simulink model "Melo"  (Simulink 6.5)
settings: Solver=FixedStepDiscrete  SolverMode=SingleTasking  StartTime=0.0  StopTime=3  RelTol=1e-3
InitFcn:
  | Ts=2e-6; load power_acdrive_init;
undefined symbols (not defined in the file): DiscIntNeverNeededParam, powergui
libraries: powerlib x13, simulink x2
Description:
  | The Model initialization function Callback automatically
  | 
  | sets the sample time  to 2e-6 sec.  and loads the initial
  | 
  | states vector xInitial. The initial state vector is saved in the
  | 
  | power_acdrive_init.mat file.
  | 
  | 
  | 
  | Check  the Initial state checkbox in the Simulation
  | 
  | parameters/Workspace I/O to start in steady state with a
  | 
  | speed of 120 rad/s and a torque of 0 N.m/s,
settings Model: Creator=Hoang Lehuy, Laval University  LastModifiedBy=RS  ExtModeTrigMode=oneshot  ExtModeArmWhenConnect=off  ExtModeAutoUpdateStatusClock=off
settings DataIOCC: LimitDataPoints=off  SaveFinalState=on  SaveOutput=off  SaveTime=off  SignalLoggingName=sigsOut
settings OptimizationCC: BlockReduction=off  InlineInvariantSignals=on
settings DebuggingCC: CheckExecutionContextPreStartOutputMsg=on  CheckExecutionContextRuntimeOutputMsg=on  SolverPrmCheckMsg=none  MultiTaskDSMMsg=warning  MultiTaskCondExecSysMsg=none  UnconnectedOutputMsg=none  StrictBusMsg=None
settings HardwareCC: TargetUnknown=on
settings RTWCC: IncludeERTFirstTime=on

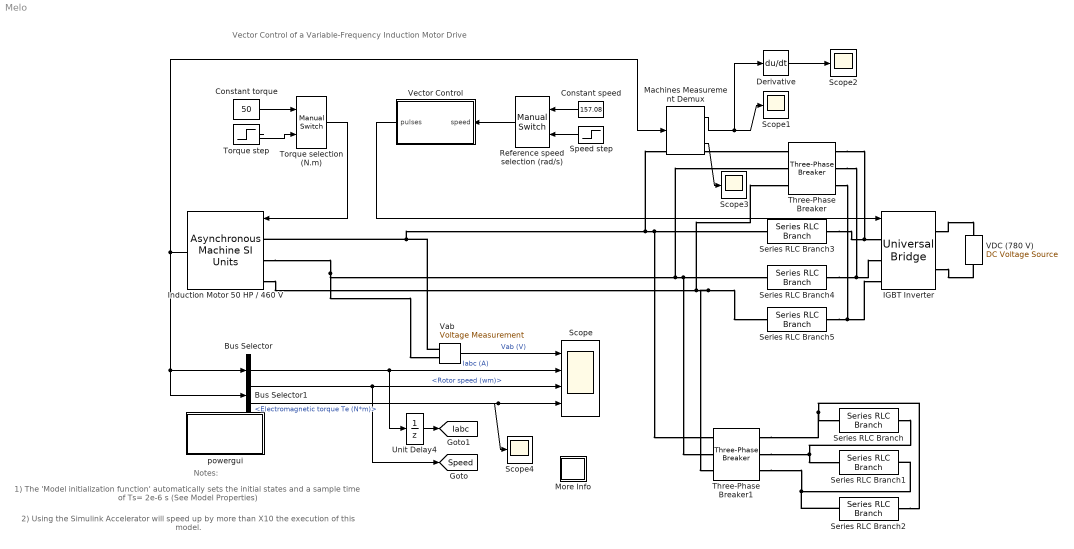
== system Melo ==
  note: Vector Control of a Variable-Frequency Induction Motor Drive
  note: 2) Using the Simulink Accelerator will speed up by more
      |      than X10 the execution of this model.
  note: 1) The 'Model initialization function' automatically sets  the initial states
      |     and a sample time of Ts= 2e-6 s  (See Model Properties)
  note: Notes:
  Bus Selector : BusSelector  OutputSignals=Stator measurements.Stator current is_a (A),Stator measurements.Stator current is_b (A),Stator measurements.Stator current is_c (A)  OutputAsBus=on
  Bus Selector1 : BusSelector  OutputSignals=Mechanical.Rotor speed (wm),Mechanical.Electromagnetic torque Te (N*m)
  Constant speed : Constant  Orientation=left  Value=157.08  OutDataType=sfix(16)  ConRadixGroup=Use specified scaling  OutScaling=2^0  SampleTime=inf  FramePeriod=inf
  Constant torque : Constant  Value=50  OutDataType=sfix(16)  ConRadixGroup=Use specified scaling  OutScaling=2^0  SampleTime=inf  FramePeriod=inf
  Derivative : Derivative
  IGBT Inverter : powerlib/Power Electronics/Universal Bridge  DialogController=PMDialogs.PMDefaultMaskDlg  SystemSampleTime=-1  Arms=3  SnubberResistance=1000  SnubberCapacitance=inf  Device=IGBT / Diodes  Ron=1e-3  Lon=0  ForwardVoltages="[  0.8  0.8  ]"  ForwardVoltage=.8  GTOparameters=[ 1e-6 , 1e-6 ]  IGBTparameters=[ 1e-6 , 2e-6 ]  Measurements=None  converterType=Rectifier
  Induction Motor 50 HP / 460 V : powerlib/Machines/Asynchronous Machine SI Units  Orientation=left  DialogController=PMDialogs.PMDefaultMaskDlg  SystemSampleTime=-1  PresetModel=No  MechanicalLoad=Torque Tm  ShowDetailedParameters=on  RotorType=Squirrel-cage  ReferenceFrame=Stationary  NominalParameters=[ 50*746, 460, 60 ]  Stator=[ 0.087 0.8e-3 ]  Rotor="[ 0.228  0.8e-3 ]"  Lm=34.7e-3  Mechanical="[1.662  0.1 2 ]"  PolePairs=2  InitialConditions="[ 1, 0 ,  0 , 0 , 0 , 0 , 0 , 0 ]"  Units=1  LoadFlowParameters=0  SimulateSaturation=off  Saturation=[0 0;0 0]
  Machines Measurement Demux : powerlib/Machines/Machines Measurement Demux  DialogController=PMDialogs.PMDefaultMaskDlg  SystemSampleTime=-1  machType=Asynchronous  ssm1=on  ssm2=on  ssm3=on  ssm4=on  ssm5=on  ssm6=on  sm1=off  sm2=off  sm3=off  sm4=off  sm5=off  sm6=off  sm7=off  sm8=on  sm9=off  sm10=off  sm11=off  sm115=off  sm12=off  sm13=off  sm14=off  asm1=off  asm2=off  asm3=off  asm4=off  asm5=off  asm6=off  asm7=on  asm8=on  asm9=off  asm10=off  asm11=off  pmsm1=on  pmsm2=on  pmsm3=on  pmsm4=off  pmsm5=on  pmsm6=on  pmsm7=on  lastType=1
  More Info : Subsystem
      settings: OpenFcn=showdemo(bdroot(gcb))
      mask Display: disp('?')
  Reference speed selection (rad/s) : simulink/Signal Routing/Manual Switch  Orientation=left  SystemSampleTime=-1  sw=1  action=0
  Scope : Scope  NumInputPorts=4
      settings: TimeRange=3  YMin=-1000~-500~0~-100  YMax=1000~500~200~400  Decimation=20  SampleTime=5e-6
  Scope{1..4} (4 alike) : Scope
      Scope1 settings: Decimation=20
      Scope2 settings: SaveName=ScopeData2  Decimation=20
      Scope3 settings: SaveName=ScopeData3  Decimation=20
      Scope4 settings: SaveName=ScopeData4  MaxDataPoints=10000000  Decimation=20
  Series RLC Branch : powerlib/Elements/Series RLC Branch  DialogController=PMDialogs.PMDefaultMaskDlg  PhysicalDomain=powersysdomain  SubClassName=unknown  LeftPortType=p1  RightPortType=p1  LConnTagsString=__new0  RConnTagsString=__new0  BranchType=C  Resistance=1  Inductance=1e-3  SetiL0=off  InitialCurrent=0  Capacitance=1e-3  Setx0=off  InitialVoltage=0  Measurements=None
  Series RLC Branch1 : powerlib/Elements/Series RLC Branch  DialogController=PMDialogs.PMDefaultMaskDlg  PhysicalDomain=powersysdomain  SubClassName=unknown  LeftPortType=p1  RightPortType=p1  LConnTagsString=__new0  RConnTagsString=__new0  BranchType=C  Resistance=1  Inductance=1e-3  SetiL0=off  InitialCurrent=0  Capacitance=1e-3  Setx0=off  InitialVoltage=0  Measurements=None
  Series RLC Branch2 : powerlib/Elements/Series RLC Branch  DialogController=PMDialogs.PMDefaultMaskDlg  PhysicalDomain=powersysdomain  SubClassName=unknown  LeftPortType=p1  RightPortType=p1  LConnTagsString=__new0  RConnTagsString=__new0  BranchType=C  Resistance=1  Inductance=1e-3  SetiL0=off  InitialCurrent=0  Capacitance=1e-3  Setx0=off  InitialVoltage=0  Measurements=None
  Series RLC Branch3 : powerlib/Elements/Series RLC Branch  DialogController=PMDialogs.PMDefaultMaskDlg  PhysicalDomain=powersysdomain  SubClassName=unknown  LeftPortType=p1  RightPortType=p1  LConnTagsString=__new0  RConnTagsString=__new0  BranchType=R  Resistance=3  Inductance=1e-3  SetiL0=off  InitialCurrent=0  Capacitance=1e-6  Setx0=off  InitialVoltage=0  Measurements=None
  Series RLC Branch4 : powerlib/Elements/Series RLC Branch  DialogController=PMDialogs.PMDefaultMaskDlg  PhysicalDomain=powersysdomain  SubClassName=unknown  LeftPortType=p1  RightPortType=p1  LConnTagsString=__new0  RConnTagsString=__new0  BranchType=R  Resistance=3  Inductance=1e-3  SetiL0=off  InitialCurrent=0  Capacitance=1e-6  Setx0=off  InitialVoltage=0  Measurements=None
  Series RLC Branch5 : powerlib/Elements/Series RLC Branch  DialogController=PMDialogs.PMDefaultMaskDlg  PhysicalDomain=powersysdomain  SubClassName=unknown  LeftPortType=p1  RightPortType=p1  LConnTagsString=__new0  RConnTagsString=__new0  BranchType=R  Resistance=3  Inductance=1e-3  SetiL0=off  InitialCurrent=0  Capacitance=1e-6  Setx0=off  InitialVoltage=0  Measurements=None
  Speed step : Step  Orientation=left  Time=0.2  Before=120  After=160  SampleTime=0
  Three-Phase Breaker : powerlib/Elements/Three-Phase Breaker  DialogController=PMDialogs.PMDefaultMaskDlg  SystemSampleTime=-1  InitialState=closed  SwitchA=on  SwitchB=on  SwitchC=on  SwitchTimes=0  External=off  BreakerResistance=0.001  SnubberResistance=1e6  SnubberCapacitance=inf  Measurements=None
  Three-Phase Breaker1 : powerlib/Elements/Three-Phase Breaker  DialogController=PMDialogs.PMDefaultMaskDlg  SystemSampleTime=-1  InitialState=open  SwitchA=on  SwitchB=on  SwitchC=on  SwitchTimes=0  External=off  BreakerResistance=0.001  SnubberResistance=1e6  SnubberCapacitance=inf  Measurements=None
  Torque selection (N.m) : simulink/Signal Routing/Manual Switch  SystemSampleTime=-1  sw=0  action=0
  Torque step : Step  Time=1.8  After=50  SampleTime=0
  Unit Delay4 : UnitDelay  SampleTime=Ts
  VDC (780 V) : powerlib/Electrical Sources/DC Voltage Source  Description=source block  Orientation=up  DialogController=PMDialogs.PMDefaultMaskDlg  SystemSampleTime=-1  Amplitude=780  Measurements=None
      settings: AttributesFormatString=\n
  Vab : powerlib/Measurements/Voltage Measurement  Tag=PoWeRsYsTeMmEaSuReMeNt  DialogController=PMDialogs.PMDefaultMaskDlg  SystemSampleTime=-1  PhasorSimulation=off  OutputType=Magnitude  PSBequivalent=0
  Vector Control : Subsystem  Orientation=left
  powergui : Subsystem  Priority=2  AncestorBlock=powerlib/powergui  InitFcn=powergui( 'InitFcn_Callback' , gcb , 0 , [ ] );  mask(PSB option menu block){SimulationMode=Discrete, SampleTime=Ts, echomessages=off, RestoreLinks=warning, x0status=blocks, Frange=[0:2:500], Ylog=off, Xlog=on, ShowGrid=off, save=off, variable=ZData, structure=ScopeData4, ZoomFFT=on, StartTime=2.8, cycles=10, DisplayStyle=2, fundamental=100, FreqAxis=off, MaxFrequency=1000, frequencyindice=60, frequencyindicesteady=1, RmsSteady=1, display=off, Ts=0, frequency=60, methode=off, HookPort=off, Interpol=off}
      mask prompts: SimulationMode "Simulation mode"; SampleTime "Sample time Ts (when simulation mode is Discrete) (s)"; echomessages "Echo  Messages"; RestoreLinks "Restore disabled links"; x0status "Initial electrical states status"; Frange "Impedance tool: Frequency Range"; Ylog "Impedance tool: Log impedance"; Xlog "Impedance tool: log Frequency"; ShowGrid "Impedance tool: grid"; save "Impedance tool: Save Data To Workspace"; variable "Impedance tool: Variable Name"; structure "Structure Name (PSBFFTSCOPE)"; ZoomFFT "ZoomFFT (PSBFFTSCOPE)"; StartTime "Start Time (PSBFFTSCOPE)"; cycles "Cycles (PSBFFTSCOPE)"; DisplayStyle "Display style (PSBFFTSCOPE)"; fundamental "Fundamental (PSBFFTSCOPE)"; FreqAxis "Frequency Axis (PSBFFTSCOPE)"; MaxFrequency "Max Frequency (PSBFFTSCOPE)"; frequencyindice "Load flow frequency (Hz)"; frequencyindicesteady "Frequency indice (STEADYSTATE)"; RmsSteady "RMS display (STEADYSTATE)"; display "Display Results"; Ts "OBSOLETE 1"; frequency "Phasor frequency (Hz)"; methode "Phasor simulation"; HookPort "Hook port"; Interpol "Interpolate"
      mask init:
      | powerlibroot = which('powersysdomain');
      | PSBroot = powerlibroot(1:end-16);
      | %
      | switch SimulationMode
      | 	case 1
      | 		message=sprintf('Continuous');
      | 	case 2
      |         SampleTimeeval=evalin('base',SampleTime,'NaN');
      |         if isnan(SampleTimeeval)
      |             message=sprintf('Warning !!,\nUndefined sample time');
      |         else
      |             message=sprintf('Discrete,\nTs = %.4g s.',SampleTimeeval);
      |         end
      | 	case 3
      | 		message=sprintf('Phasors');
      | end
      | if strcmp(bdroot,'powerlib')
      |   message='powergui';
      | end
      | power_initmask();
      settings: CopyFcn=powergui( 'Copy_Callback' , gcb , 0 , [ ] );  ModelCloseFcn=powergui( 'CloseButton_Callback' , gcb , [ ] , [ ] );  PreSaveFcn=powergui( 'CloseButton_Callback' , gcb , [ ] , [ ] );  NameChangeFcn=powergui( 'NameChangeFcn_Callback' , gcb , 0 , [ ] );
      settings: DeleteFcn=|
      | powergui( 'Copy_Callback' , gcb , 1 , [ ] );
      | powergui( 'CloseButton_Callback' , gcb , [ ] , [ ] );
      settings: OpenFcn=|
      | if (power_openblockproxy ('secondary'))
      | powergui(gcb,'PM')
      | end;
      mask Help: web(psbhelp)
      mask StyleString: popup(Continuous|Discrete|Phasor),edit,checkbox,popup(yes|warning|no),popup(blocks|steady|zero),edit,checkbox,checkbox,checkbox,checkbox,edit,edit,checkbox,edit,edit,edit,edit,checkbox,edit,edit,edit,edit,checkbox,edit,edit,checkbox,checkbox,checkbox
      mask CallbackString: ||||||||||||||||||||||||||powergui('HookPort',[],[],gcb);|
      mask Display: disp(message)
  tag scope: Iabc=global, Speed=global
  wires:
  Bus Selector1/1 -> Scope/3, [Speed]  "<Rotor speed (wm)>"
  Vector Control/1(pulses) -> IGBT Inverter/1
  Torque step/1 -> Torque selection (N.m)/2
  Constant torque/1 -> Torque selection (N.m)/1
  Constant speed/1 -> Reference speed selection (rad/s)/1
  Speed step/1 -> Reference speed selection (rad/s)/2
  Bus Selector/1 -> Scope/2, Unit Delay4/1  "Iabc (A)"
  Vab/1 -> Scope/1  "Vab (V)"
  Bus Selector1/2 -> Scope/4, Scope4/1  "<Electromagnetic torque Te (N*m)>"
  Torque selection (N.m)/1 -> Induction Motor 50 HP / 460 V/1
  Reference speed selection (rad/s)/1 -> Vector Control/1(speed)
  Induction Motor 50 HP / 460 V/1 -> Bus Selector1/1, Bus Selector/1, Machines Measurement Demux/1
  Unit Delay4/1 -> [Iabc]
  Machines Measurement Demux/1 -> Scope1/1, Derivative/1
  Derivative/1 -> Scope2/1
  Machines Measurement Demux/2 -> Scope3/1
  connections:
  IGBT Inverter/RConn2 -- VDC (780 V)/LConn1
  IGBT Inverter/RConn1 -- VDC (780 V)/RConn1
  Series RLC Branch/RConn1 -- Series RLC Branch1/LConn1 -- Three-Phase Breaker1/RConn2
  Series RLC Branch2/RConn1 -- Series RLC Branch/LConn1 -- Three-Phase Breaker1/RConn1
  Series RLC Branch4/RConn1 -- IGBT Inverter/LConn2 -- Three-Phase Breaker/RConn2
  Series RLC Branch2/LConn1 -- Series RLC Branch1/RConn1 -- Three-Phase Breaker1/RConn3
  Vab/LConn1 -- Induction Motor 50 HP / 460 V/LConn1 -- Three-Phase Breaker/LConn1 -- Series RLC Branch3/LConn1 -- Three-Phase Breaker1/LConn1
  Induction Motor 50 HP / 460 V/LConn2 -- Vab/LConn2 -- Three-Phase Breaker/LConn2 -- Series RLC Branch4/LConn1 -- Three-Phase Breaker1/LConn2
  Induction Motor 50 HP / 460 V/LConn3 -- Three-Phase Breaker/LConn3 -- Series RLC Branch5/LConn1 -- Three-Phase Breaker1/LConn3
  Series RLC Branch5/RConn1 -- IGBT Inverter/LConn3 -- Three-Phase Breaker/RConn3
  Series RLC Branch3/RConn1 -- IGBT Inverter/LConn1 -- Three-Phase Breaker/RConn1

== system Melo/More Info ==
  note: H. Le-Huy (Universite Laval, Quebec)
  note: Case study : Variable-Frequency Induction Motor Drive
  note: Circuit Description
  note: Demonstration
  note: The induction motor is fed by a current-controlled PWM inverter which is built using a Universal Bridge block.
      | The motor drives a mechanical load characterized by inertia J, friction coeficient B, and load torque TL .
      | The speed control loop uses a proportional-integral controller to produce the quadrature-axis current reference
      | iq* which controls the motor torque.  The motor flux is controlled by the direct-axis current reference id*.
      | Block DQ-ABC is used to convert id* and iq* into current references ia*, ib*, and ic* for the current regulator.
      | Current and Voltage Measurement blocks provide signals for visualization purpose.
      | Motor current, speed, and torque signals are available at the output of the 'Asynchronous Machine' block.
  note: Motor starting
  note: Start the simulation. Observe the motor current, voltage, and speed during the starting on the scope.
      | At the end of the simulation time (3 s), the system has reached its steady-state.
  note: Response to a change in reference speed and load torque
  note: The initial conditions state vector `xInitial' to start with wm = 120 rad/s and TL = 0 N.m has been saved in the 'power_acdrive_init.mat'  file.
      | This file is automatically loaded in your  workspace when you start the simulation (see  Model Properties).
      | In order to use these initial conditions you have to enable them. Check the Simulation/Configuration Parameters menu ,
      | then select "Data Import/Export" and check "Initial state".
      |
      | Now, double click the two Manual Switch blocks to switch from  the  "Constant speed " and  "Constant torque" blocks to the Step blocks.
      | (Reference speed wref changed from 120 to 160 rad/s at t = 0.2 s and load torque changed from 0 to 200 N.m at  t= 1.8s).
      | Restart the simulation  and observe the drive response to successive changes in speed reference and load torque.

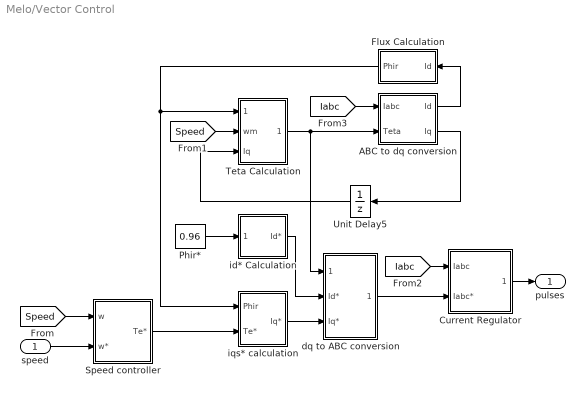
== system Melo/Vector Control ==
  speed : Inport
  ABC to dq conversion : Subsystem
  Current Regulator : Subsystem  mask(Regulateur de courant a hysteresis){h=20}
      mask prompts: h "Hysteresis band (A)"
  Flux Calculation : Subsystem  Orientation=left  mask(Flux Calcultation){}
      mask init:
      | NF=0.44572610323020e-6;
      | DF=[1 -0.99998715486734];
  Phir* : Constant  Value=0.96  OutDataType=sfix(16)  ConRadixGroup=Use specified scaling  OutScaling=2^0  SampleTime=inf  FramePeriod=inf
  Speed controller : Subsystem  mask(PI controller){Kp=13, Ki=26, Tlim=300, Ts=Ts}
      mask prompts: Kp "Proportional gain (Kp)"; Ki "Integral gain (Ki)"; Tlim "Torque limit (N.m)"; Ts "Sampling time (s)"
      mask help: Proportional-Integral Speed Controller
      mask Display: plot(0,0,100,100,[35,35,65],[70,30,30],[35,65],[45,60])
  Teta Calculation : Subsystem
  Unit Delay5 : UnitDelay  Orientation=left  SampleTime=Ts
  dq to ABC conversion : Subsystem
  id* Calculation : Subsystem
  iqs* calculation : Subsystem
  pulses : Outport
  wires:
  dq to ABC conversion/1(Iabc*) -> Current Regulator/2(Iabc*)
  Speed controller/1(Te*) -> iqs* calculation/2(Te*)
  Phir*/1 -> id* Calculation/1(Phir*)
  ABC to dq conversion/1(Id) -> Flux Calculation/1(Id)
  id* Calculation/1(Id*) -> dq to ABC conversion/2(Id*)
  Flux Calculation/1(Phir) -> Teta Calculation/1(Phir), iqs* calculation/1(Phir)
  ABC to dq conversion/2(Iq) -> Unit Delay5/1
  Unit Delay5/1 -> Teta Calculation/3(Iq)
  iqs* calculation/1(Iq*) -> dq to ABC conversion/3(Iq*)
  Teta Calculation/1(Teta) -> dq to ABC conversion/1(Teta), ABC to dq conversion/2(Teta)
  [Speed] -> Speed controller/1(w)
  [Speed] -> Teta Calculation/2(wm)
  [Iabc] -> Current Regulator/1(Iabc)
  [Iabc] -> ABC to dq conversion/1(Iabc)
  speed/1 -> Speed controller/2(w*)
  Current Regulator/1(Pulses) -> pulses/1

== system Melo/powergui ==
  note: Graphical user interface for the analysis of  SimPowerSystems circuits.
      | Place the Powergui block in the top-level of your model and double-click
      | on it to open the GUI.
  EquivalentModel1 : Subsystem
      mask init:
      | SPS = get_param(gcbh,'UserData');
      | if isempty(SPS)
      | 	Ts=1;
      |     A=0;
      |     B=0;
      |     C=0;
      |     D=0;
      |     x0=0;
      |     SwitchResistance=1;
      |     SwitchType=1;
      |     SwitchGateInitialValue=1;
      |     OutputsToResetToZero=1;
      | else
      | 	Ts=SPS.PowerguiInfo.Ts;
      | 	A=SPS.Adiscrete;
      |     B=SPS.Bdiscrete;
      |     C=SPS.Cdiscrete;
      |     D=SPS.Ddiscrete;
      |     x0=SPS.x0discrete;
      |     SwitchResistance=SPS.SwitchResistance;
      |     SwitchType=SPS.SwitchType;
      |     SwitchGateInitialValue=SPS.SwitchGateInitialValue;
      |     OutputsToResetToZero=SPS.YSwitchCurrent;
      | end
      mask Display:
      | color('orange')
      | disp('EQUIVALENT CIRCUIT')
  Ground : Ground
  Terminator : Terminator
  wires:
  Ground/1 -> Terminator/1

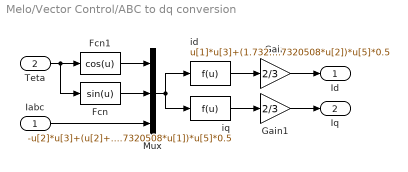
== system Melo/Vector Control/ABC to dq conversion ==
  Iabc : Inport
  Teta : Inport  Port=2
  Fcn : Fcn  Expr=sin(u)
  Fcn1 : Fcn  Expr=cos(u)
  Gain : Gain  Gain=2/3  SaturateOnIntegerOverflow=on
  Gain1 : Gain  Gain=2/3  SaturateOnIntegerOverflow=on
  Mux : Mux  Inputs=[1 1 3]
  id : Fcn  Expr=u[1]*u[3]+(1.7320508*u[2]-u[1])*u[4]*0.5+(-u[1]-1.7320508*u[2])*u[5]*0.5
  iq : Fcn  Expr=-u[2]*u[3]+(u[2]+1.7320508*u[1])*u[4]*0.5+(u[2]-1.7320508*u[1])*u[5]*0.5
  Id : Outport  InitialOutput=0
  Iq : Outport  Port=2  InitialOutput=0
  wires:
  Fcn/1 -> Mux/2
  Fcn1/1 -> Mux/1
  Teta/1 -> Fcn1/1, Fcn/1
  Mux/1 -> iq/1, id/1
  Iabc/1 -> Mux/3
  iq/1 -> Gain1/1
  id/1 -> Gain/1
  Gain/1 -> Id/1
  Gain1/1 -> Iq/1

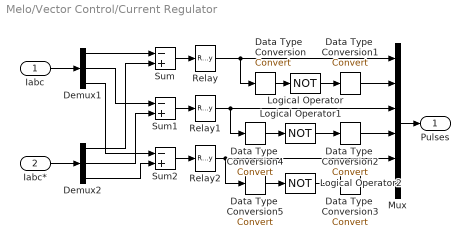
== system Melo/Vector Control/Current Regulator ==
  Iabc : Inport
  Iabc* : Inport  Port=2
  Data Type  Conversion : DataTypeConversion  OutDataTypeMode=boolean  SaturateOnIntegerOverflow=on  RndMeth=Zero
  Data Type  Conversion1 : DataTypeConversion  OutDataTypeMode=double  SaturateOnIntegerOverflow=on  RndMeth=Zero
  Data Type  Conversion2 : DataTypeConversion  OutDataTypeMode=double  SaturateOnIntegerOverflow=on  RndMeth=Zero
  Data Type  Conversion3 : DataTypeConversion  OutDataTypeMode=double  SaturateOnIntegerOverflow=on  RndMeth=Zero
  Data Type  Conversion4 : DataTypeConversion  OutDataTypeMode=boolean  SaturateOnIntegerOverflow=on  RndMeth=Zero
  Data Type  Conversion5 : DataTypeConversion  OutDataTypeMode=boolean  SaturateOnIntegerOverflow=on  RndMeth=Zero
  Demux1 : Demux  Outputs=3
  Demux2 : Demux  Outputs=3
  Logical Operator : Logic  Operator=NOT
  Logical Operator1 : Logic  Operator=NOT
  Logical Operator2 : Logic  Operator=NOT
  Mux : Mux  Inputs=6
  Relay : Relay  OnSwitchValue=h/2  OffSwitchValue=-h/2
  Relay1 : Relay  OnSwitchValue=h/2  OffSwitchValue=-h/2
  Relay2 : Relay  OnSwitchValue=h/2  OffSwitchValue=-h/2
  Sum : Sum  Inputs=-+  SaturateOnIntegerOverflow=on  InputSameDT=on
  Sum1 : Sum  Inputs=-+  SaturateOnIntegerOverflow=on  InputSameDT=on
  Sum2 : Sum  Inputs=-+  SaturateOnIntegerOverflow=on  InputSameDT=on
  Pulses : Outport  InitialOutput=0
  wires:
  Sum/1 -> Relay/1
  Sum1/1 -> Relay1/1
  Demux1/1 -> Sum/1
  Demux1/2 -> Sum1/1
  Mux/1 -> Pulses/1
  Iabc/1 -> Demux1/1
  Sum2/1 -> Relay2/1
  Demux1/3 -> Sum2/1
  Demux2/3 -> Sum2/2
  Demux2/2 -> Sum1/2
  Demux2/1 -> Sum/2
  Iabc*/1 -> Demux2/1
  Relay/1 -> Mux/1, Data Type  Conversion/1
  Relay1/1 -> Mux/3, Data Type  Conversion4/1
  Relay2/1 -> Mux/5, Data Type  Conversion5/1
  Data Type  Conversion/1 -> Logical Operator/1
  Logical Operator/1 -> Data Type  Conversion1/1
  Data Type  Conversion1/1 -> Mux/2
  Logical Operator1/1 -> Data Type  Conversion2/1
  Data Type  Conversion2/1 -> Mux/4
  Logical Operator2/1 -> Data Type  Conversion3/1
  Data Type  Conversion3/1 -> Mux/6
  Data Type  Conversion4/1 -> Logical Operator1/1
  Data Type  Conversion5/1 -> Logical Operator2/1

== system Melo/Vector Control/Flux Calculation ==
  note: Phir = Lm *Id / (1 +Tr .s)
  note: Lm = 34.7 mH
  note: Lr = Ll'r +Lm = 0.8 +34.7= 35.5 mH
  note: Tr = Lr / Rr = 0.1557 s
  note: Rr = 0.228 ohms
  Id : Inport  Orientation=left
  Discrete Tranfer Function : Subsystem  Orientation=left  mask(First Order Low Pass Filter (Discrete)){T=0.1557, Ts=Ts}
      mask prompts: T "Time constant T (s) :"; Ts "Time step (s)"
      mask help: H(s)=1/(1+T.s)
      mask init:
      | X=[0 1 2 3 4];
      |  Y=[-2 -2 -3 -4 -4];
      |  str=sprintf('\nH=1/(1+T.s)\n T= %g s\n\n\n',T);
      | num=1;
      | den=[T 1];
      | 
      | % discrete transfer function
      | % descending powers of z
      | numd= Ts/T;
      | dend=[ 1  (Ts-T)/T];
      mask Display:
      | plot(X,Y);
      | disp(str);
  Lm : Gain  Orientation=left  Gain=34.7e-3  SaturateOnIntegerOverflow=on
  Phir : Outport  Orientation=left
  wires:
  Discrete Tranfer Function/1(Out) -> Phir/1
  Id/1 -> Lm/1
  Lm/1 -> Discrete Tranfer Function/1(In)

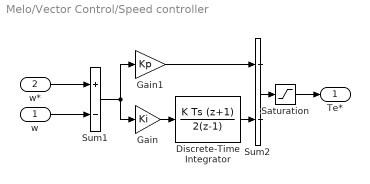
== system Melo/Vector Control/Speed controller ==
  w : Inport
  w* : Inport  Port=2
  Discrete-Time Integrator : DiscreteIntegrator  IntegratorMethod=Integration: Trapezoidal  SampleTime=Ts  LimitOutput=on  UpperSaturationLimit=Tlim  LowerSaturationLimit=-Tlim  ICPrevOutput=DiscIntNeverNeededParam  ICPrevScaledInput=DiscIntNeverNeededParam
  Gain : Gain  Gain=Ki  SaturateOnIntegerOverflow=on
  Gain1 : Gain  Gain=Kp  SaturateOnIntegerOverflow=on
  Saturation : Saturate  UpperLimit=Tlim  LowerLimit=-Tlim
  Sum1 : Sum  Inputs=+-  SaturateOnIntegerOverflow=on  InputSameDT=on
  Sum2 : Sum  SaturateOnIntegerOverflow=on  InputSameDT=on
  Te* : Outport  InitialOutput=0
  wires:
  Gain1/1 -> Sum2/1
  Gain/1 -> Discrete-Time Integrator/1
  Sum1/1 -> Gain/1, Gain1/1
  Discrete-Time Integrator/1 -> Sum2/2
  Sum2/1 -> Saturation/1
  Saturation/1 -> Te*/1
  w/1 -> Sum1/2
  w*/1 -> Sum1/1

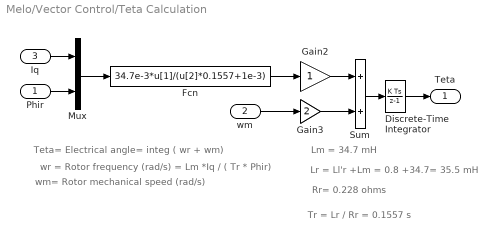
== system Melo/Vector Control/Teta Calculation ==
  note: Teta= Electrical angle= integ ( wr + wm)
  note: wr = Rotor frequency (rad/s) = Lm *Iq / ( Tr * Phir)
  note: Lm = 34.7 mH
  note: Rr= 0.228 ohms
  note: Lr = Ll'r +Lm = 0.8 +34.7= 35.5 mH
  note: wm= Rotor mechanical speed (rad/s)
  note: Tr = Lr / Rr = 0.1557 s
  Phir : Inport
  wm : Inport  Port=2
  Iq : Inport  Port=3
  Discrete-Time Integrator : DiscreteIntegrator  SampleTime=Ts  ICPrevOutput=DiscIntNeverNeededParam  ICPrevScaledInput=DiscIntNeverNeededParam
  Fcn : Fcn  Expr=34.7e-3*u[1]/(u[2]*0.1557+1e-3)
  Gain2 : Gain  SaturateOnIntegerOverflow=on
  Gain3 : Gain  Gain=2  SaturateOnIntegerOverflow=on
  Mux : Mux  Inputs=2
  Sum : Sum  SaturateOnIntegerOverflow=on  InputSameDT=on
  Teta : Outport  InitialOutput=0
  wires:
  Discrete-Time Integrator/1 -> Teta/1
  Sum/1 -> Discrete-Time Integrator/1
  Gain3/1 -> Sum/2
  Gain2/1 -> Sum/1
  wm/1 -> Gain3/1
  Fcn/1 -> Gain2/1
  Phir/1 -> Mux/2
  Iq/1 -> Mux/1
  Mux/1 -> Fcn/1

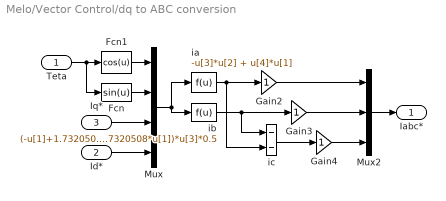
== system Melo/Vector Control/dq to ABC conversion ==
  Teta : Inport
  Id* : Inport  Port=2
  Iq* : Inport  Port=3
  Fcn : Fcn  Expr=sin(u)
  Fcn1 : Fcn  Expr=cos(u)
  Gain2 : Gain  SaturateOnIntegerOverflow=on
  Gain3 : Gain  SaturateOnIntegerOverflow=on
  Gain4 : Gain  SaturateOnIntegerOverflow=on
  Mux : Mux
  Mux2 : Mux  Inputs=3
  ia : Fcn  Expr=-u[3]*u[2] + u[4]*u[1]
  ib : Fcn  Expr=(-u[1]+1.7320508*u[2])*u[4]*0.5+(u[2]+1.7320508*u[1])*u[3]*0.5
  ic : Sum  Inputs=--  SaturateOnIntegerOverflow=on  InputSameDT=on
  Iabc* : Outport  InitialOutput=0
  wires:
  Fcn/1 -> Mux/2
  Fcn1/1 -> Mux/1
  Mux2/1 -> Iabc*/1
  Mux/1 -> ib/1, ia/1
  Teta/1 -> Fcn1/1, Fcn/1
  Iq*/1 -> Mux/3
  Id*/1 -> Mux/4
  Gain3/1 -> Mux2/2
  ic/1 -> Gain4/1
  Gain4/1 -> Mux2/3
  Gain2/1 -> Mux2/1
  ia/1 -> Gain2/1, ic/2
  ib/1 -> Gain3/1, ic/1

== system Melo/Vector Control/id* Calculation ==
  note: Id* = Phir*/ Lm
  note: Lm= 34.7 mH
  Phir* : Inport
  KF : Gain  Gain=1/34.7e-3  SaturateOnIntegerOverflow=on
  Id* : Outport
  wires:
  KF/1 -> Id*/1
  Phir*/1 -> KF/1

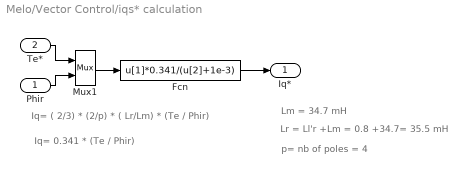
== system Melo/Vector Control/iqs* calculation ==
  note: Iq= ( 2/3) * (2/p) * ( Lr/Lm) * (Te / Phir)
  note: Lm = 34.7 mH
  note: Lr = Ll'r +Lm = 0.8 +34.7= 35.5 mH
  note: p= nb of poles = 4
  note: Iq= 0.341 * (Te / Phir)
  Phir : Inport
  Te* : Inport  Port=2
  Fcn : Fcn  Expr=u[1]*0.341/(u[2]+1e-3)
  Mux1 : Mux  Inputs=2
  Iq* : Outport  InitialOutput=0
  wires:
  Phir/1 -> Mux1/2
  Fcn/1 -> Iq*/1
  Te*/1 -> Mux1/1
  Mux1/1 -> Fcn/1

== system Melo/powergui/EquivalentModel1 ==
  Gates : Subsystem
  Sources : Subsystem
  State-Space : S-Function  FunctionName=sfun_spssw_discc  Parameters=Ts,A, B, C, D, x0, SwitchResistance ,SwitchType, SwitchGateInitialValue, OutputsToResetToZero
  Status : Subsystem
  Yout : Subsystem
  wires:
  State-Space/1 -> Yout/1(v,i)
  State-Space/2 -> Status/1(status)
  Sources/1(u) -> State-Space/1
  Gates/1(gates) -> State-Space/2

== system Melo/Vector Control/Flux Calculation/Discrete Tranfer Function ==
  In : Inport
  Discrete Transfer Fcn : DiscreteTransferFcn  Numerator=numd  Denominator=dend  SampleTime=Ts
  Out : Outport  InitialOutput=0
  wires:
  Discrete Transfer Fcn/1 -> Out/1
  In/1 -> Discrete Transfer Fcn/1

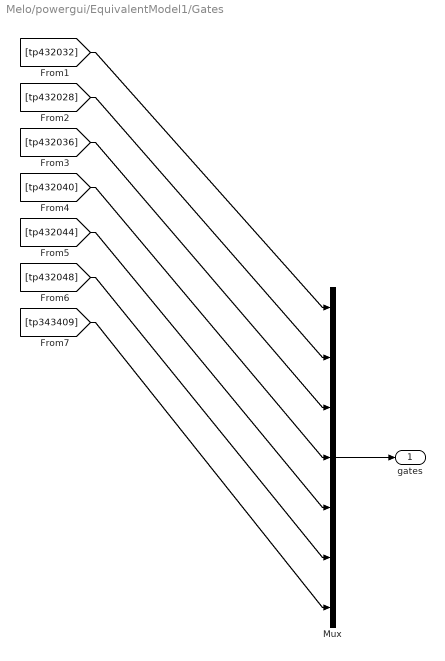
== system Melo/powergui/EquivalentModel1/Gates ==
  Mux : Mux  Inputs=[1 1 1 1 1 1 6]
  gates : Outport
  wires:
  Mux/1 -> gates/1
  [tp432032] -> Mux/1
  [tp432028] -> Mux/2
  [tp432036] -> Mux/3
  [tp432040] -> Mux/4
  [tp432044] -> Mux/5
  [tp432048] -> Mux/6
  [tp343409] -> Mux/7

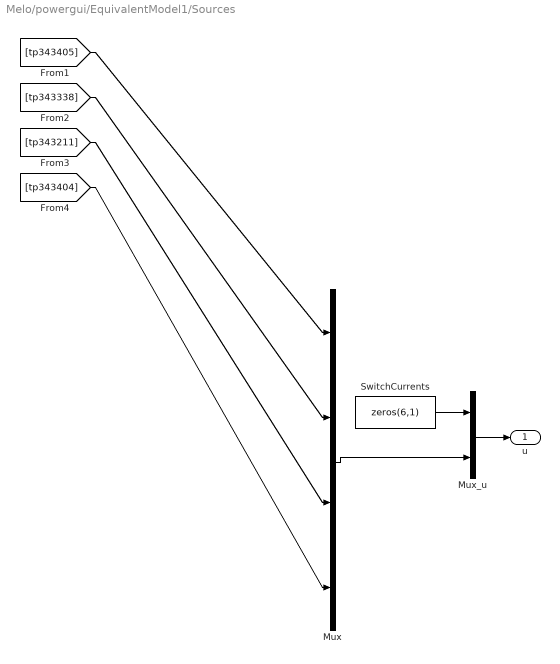
== system Melo/powergui/EquivalentModel1/Sources ==
  Mux : Mux  Inputs=[6 2 1 6]
  Mux_u : Mux  Inputs=[6 15]
  SwitchCurrents : Constant  Value=zeros(6,1)  OutDataType=sfix(16)  ConRadixGroup=Use specified scaling  OutScaling=2^0  SampleTime=inf  FramePeriod=inf
  u : Outport
  wires:
  Mux/1 -> Mux_u/2
  SwitchCurrents/1 -> Mux_u/1
  Mux_u/1 -> u/1
  [tp343405] -> Mux/1
  [tp343338] -> Mux/2
  [tp343211] -> Mux/3
  [tp343404] -> Mux/4

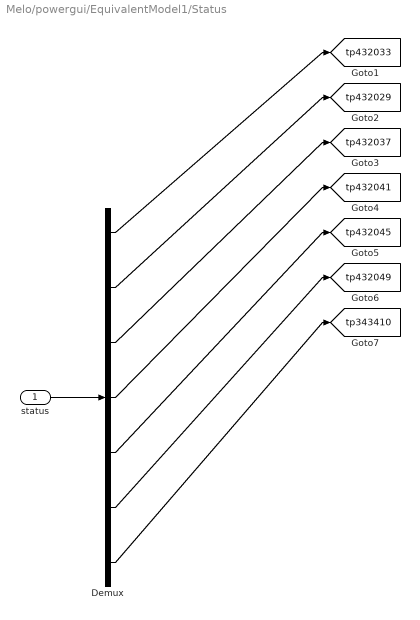
== system Melo/powergui/EquivalentModel1/Status ==
  status : Inport
  Demux : Demux  Outputs=[1 1 1 1 1 1 6]
  tag scope: tp343410=global, tp432029=global, tp432033=global, tp432037=global, tp432041=global, tp432045=global, tp432049=global
  wires:
  status/1 -> Demux/1
  Demux/1 -> [tp432033]
  Demux/2 -> [tp432029]
  Demux/3 -> [tp432037]
  Demux/4 -> [tp432041]
  Demux/5 -> [tp432045]
  Demux/6 -> [tp432049]
  Demux/7 -> [tp343410]

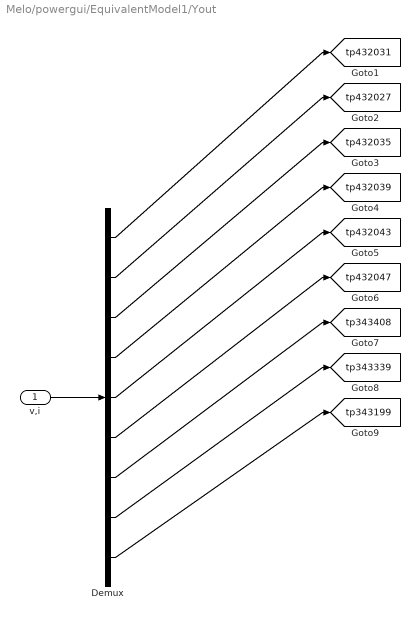
== system Melo/powergui/EquivalentModel1/Yout ==
  v,i : Inport
  Demux : Demux  Outputs=[1 1 1 1 1 1 6 2 1]
  tag scope: tp343199=global, tp343339=global, tp343408=global, tp432027=global, tp432031=global, tp432035=global, tp432039=global, tp432043=global, tp432047=global
  wires:
  v,i/1 -> Demux/1
  Demux/1 -> [tp432031]
  Demux/2 -> [tp432027]
  Demux/3 -> [tp432035]
  Demux/4 -> [tp432039]
  Demux/5 -> [tp432043]
  Demux/6 -> [tp432047]
  Demux/7 -> [tp343408]
  Demux/8 -> [tp343339]
  Demux/9 -> [tp343199]
